simulink model "MOD1"  (R2017a)
settings: Solver=ode5  StartTime=0.0  StopTime=1.0  RelTol=1e-3
undefined symbols (not defined in the file): a, b, DiscIntNeverNeededParam
libraries: dspmlti4 x3, dsparch4 x1
settings Model: Creator=bhannigan  LastModifiedBy=bhannigan
settings OptimizationCC: LifeSpan=inf
settings DebuggingCC: SFUnexpectedBacktrackingDiag=warning  SFNoUnconditionalDefaultTransitionDiag=warning  SFExecutionAtInitializationDiag=none
settings GRTTargetCC: TargetLangStandard=C89/C90 (ANSI)  GeneratePreprocessorConditionals=Disable all
settings ConfigComp: CovMetricSettings=dw  CovHtmlReporting=on  CovSaveCumulativeToWorkspaceVar=on  CovSaveSingleToWorkspaceVar=on  CovExternalEMLEnable=off

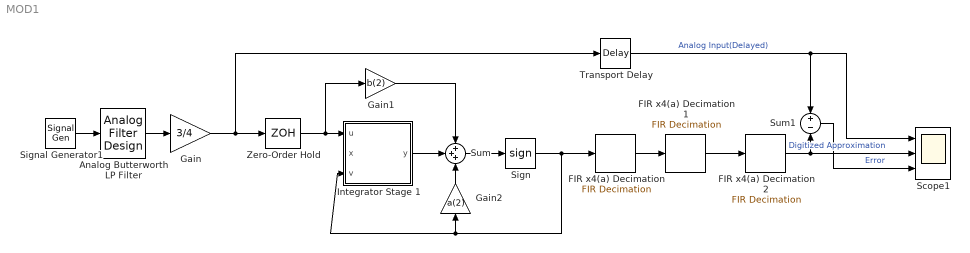
== system MOD1 ==
  Analog Butterworth LP Filter : dsparch4/Analog Filter Design  method=Butterworth  filttype=Lowpass  N=5  Wlo=2*pi*4000  Whi=80  Rp=2  Rs=40
  FIR x4(a) Decimation : dspmlti4/FIR Decimation  FilterSource=Dialog parameters  h=fir1(31,0.15)  D=4  filtStruct=Direct form  FilterObject=Hm_firdecim  framing=Allow multirate processing  inputOffset=0  outputBufInitCond=0  roundingMode=Floor  overflowMode=off  firstCoeffDataTypeStr=Inherit: Same word length as input  firstCoeffMin=[]  firstCoeffMax=[]  firstCoeffLastDataTypeStr=Inherit: Same word length as input  accumDataTypeStr=Inherit: Same as product output  accumLastDataTypeStr=Inherit: Same as product output  outputMin=[]  outputMax=[]
  FIR x4(a) Decimation1 : dspmlti4/FIR Decimation  FilterSource=Dialog parameters  h=fir1(31,0.15)  D=4  filtStruct=Direct form  FilterObject=Hm_firdecim  framing=Allow multirate processing  inputOffset=0  outputBufInitCond=0  roundingMode=Floor  overflowMode=off  firstCoeffDataTypeStr=Inherit: Same word length as input  firstCoeffMin=[]  firstCoeffMax=[]  firstCoeffLastDataTypeStr=Inherit: Same word length as input  accumDataTypeStr=Inherit: Same as product output  accumLastDataTypeStr=Inherit: Same as product output  outputMin=[]  outputMax=[]
  FIR x4(a) Decimation2 : dspmlti4/FIR Decimation  FilterSource=Dialog parameters  h=fir1(31,0.15)  D=4  filtStruct=Direct form  FilterObject=Hm_firdecim  framing=Allow multirate processing  inputOffset=0  outputBufInitCond=0  roundingMode=Floor  overflowMode=off  firstCoeffDataTypeStr=Inherit: Same word length as input  firstCoeffMin=[]  firstCoeffMax=[]  firstCoeffLastDataTypeStr=Inherit: Same word length as input  accumDataTypeStr=Inherit: Same as product output  accumLastDataTypeStr=Inherit: Same as product output  outputMin=[]  outputMax=[]
  Gain : Gain  Gain=3/4  SaturateOnIntegerOverflow=on  OutDataTypeStr=Inherit: Same as input  ParamDataTypeStr=Inherit: Same as input
  Gain1 : Gain  Gain=b(2)
  Gain2 : Gain  Gain=a(2)
  Integrator Stage 1 : Subsystem  mask{a=a(1), b=b(1)}
      mask prompts: a "Feedback gain:"; b "Feedforward gain:"
  Scope1 : Scope  NumInputPorts=3
  Sign : Signum
  Signal Generator1 : SignalGenerator  WaveForm=square  Frequency=80
  Sum : Sum  Inputs=+++
  Sum1 : Sum  Inputs=+-  SaturateOnIntegerOverflow=on  InputSameDT=on  OutDataTypeStr=Inherit: Same as first input
  Transport Delay : TransportDelay  DelayTime=336/512000
  Zero-Order Hold : ZeroOrderHold  SampleTime=1/512000
  wires:
  Gain/1 -> Transport Delay/1, Zero-Order Hold/1
  Sum/1 -> Sign/1
  Integrator Stage 1/1(y) -> Sum/2
  Gain1/1 -> Sum/1
  Sign/1 -> FIR x4(a) Decimation/1, Gain2/1, Integrator Stage 1/3(v)
  Sum1/1 -> Scope1/3  "Error"
  Zero-Order Hold/1 -> Gain1/1, Integrator Stage 1/1(u)
  Transport Delay/1 -> Sum1/1, Scope1/1  "Analog Input(Delayed)"
  Gain2/1 -> Sum/3
  FIR x4(a) Decimation/1 -> FIR x4(a) Decimation1/1
  FIR x4(a) Decimation1/1 -> FIR x4(a) Decimation2/1
  FIR x4(a) Decimation2/1 -> Scope1/2, Sum1/2  "Digitized Approximation"
  Analog Butterworth LP Filter/1 -> Gain/1
  Signal Generator1/1 -> Analog Butterworth LP Filter/1

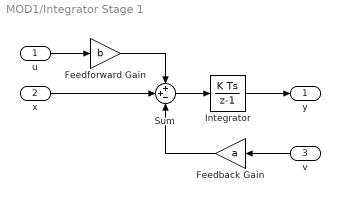
== system MOD1/Integrator Stage 1 ==
  u : Inport
  x : Inport  Port=2
  v : Inport  Port=3
  Feedback Gain : Gain  Gain=a
  Feedforward Gain : Gain  Gain=b
  Integrator : DiscreteIntegrator  InitialConditionSetting=State (most efficient)  SampleTime=-1  ICPrevOutput=DiscIntNeverNeededParam  ICPrevScaledInput=DiscIntNeverNeededParam
  Sum : Sum  Inputs=++-
  y : Outport
  wires:
  x/1 -> Sum/2
  Sum/1 -> Integrator/1
  Feedback Gain/1 -> Sum/3
  Feedforward Gain/1 -> Sum/1
  u/1 -> Feedforward Gain/1
  Integrator/1 -> y/1
  v/1 -> Feedback Gain/1
